simulink subsystem "generator_ss"  (R2022a)
settings: Solver=VariableStepAuto  StartTime=0.0  StopTime=10.0  RelTol=1e-3
model mask{obj=slPart}
  mask prompts: obj "slPart Object:"
libraries: fl_lib x2, sdl_lib x1, nesl_utility x1
settings Model: Creator=grouleau  LastModifiedBy=grouleau

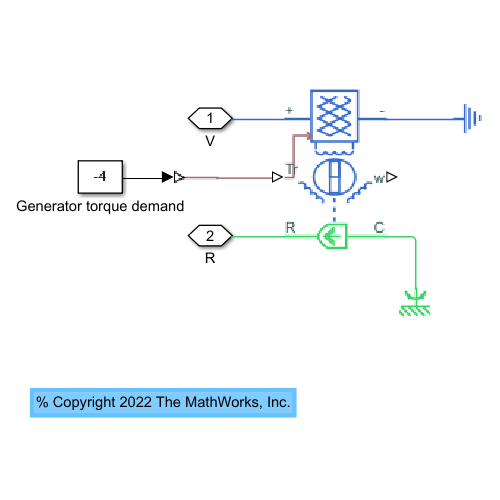
[thumbnail: Simulink's stored preview of the top-level diagram]
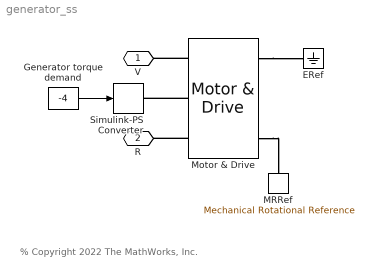
== system generator_ss ==
  note: % Copyright 2022 The MathWorks, Inc.
  ERef : fl_lib/Electrical/Electrical Elements/Electrical Reference
  Generator torque demand : Constant  Value=-4
  MRRef : fl_lib/Mechanical/Rotational Elements/Mechanical Rotational Reference
  Motor & Drive : sdl_lib/Engines & Motors/Motor & Drive  torque_max=400 N*m  power_max=obj.MaximumPower kW  Tc=0.2 s  eff=obj.Efficiency  w_eff=600 rpm  T_eff=300 N*m  thermal_port=simscape.enum.thermaleffects.omit  thermal_mass=100 J/K  temperature_specify=off  temperature_priority=High  temperature=300 K  temperature_nominal_specify=off  temperature_nominal_unit=K  temperature_nominal_value=1
      settings: SourceProductBaseCode=LD  InternalSimscapePortConfiguration="{\"Bottom\":[],\"Left\":[{\"id\":\"Vp\",\"label\":\"+\",\"type\":\"foundation.electrical.electrical\"},{\"id\":\"Tr\",\"label\":\"Tr\",\"type\":\"input\"},{\"id\":\"R\",\"label\":\"R\",\"type\":\"foundation.mechanical.rotational.rotational\"}],\"Right\":[{\"id\":\"Vm\",\"label\":\"-\",\"type\":\"foundation.electrical.electrical\"},{\"id\":\"Omega\",\"label\":\"w\",\"type\":\"output\"},{\"id\":\"C\",\"label\":\"C\",\"type\":\"foundation.mechanical.rotational.rotational\"}],\"Top\":[]}"
  Simulink-PS Converter : nesl_utility/Simulink-PS Converter  PhysicalDomain=network_engine_domain  SubClassName=ps_input  LeftPortType=input  RightPortType=output  PseudoPeriodic=off  Frequencies=[]  NoiseDistribution=none  NoiseParameters=[]  Unit=N*m  AffineConversion=off  FilteringAndDerivatives=zero  SimscapeFilterOrder=1  InputFilterTimeConstant=.001  UdotUserProvided=0
      settings: SourceProductBaseCode=PW,SS
  V : PMIOPort  Side=Right
  R : PMIOPort  Port=2  Side=Left
  wires:
  Generator torque demand/1 -> Simulink-PS Converter/1
  connections:
  Motor & Drive/LConn3 -- R/RConn1
  Motor & Drive/LConn2 -- Simulink-PS Converter/RConn1
  Motor & Drive/RConn3 -- MRRef/LConn1
  Motor & Drive/RConn1 -- ERef/LConn1
  Motor & Drive/LConn1 -- V/RConn1
